simulink model "ActiveBrakeSystem"  (R2024b)
settings: Solver=VariableStepAuto  StartTime=0.0  StopTime=10  RelTol=1e-2
undefined symbols (not defined in the file or in its folder): Kd, Ki, Kp
libraries: fl_lib x24, nesl_utility x6, spsPWMGeneratorDCDCLib x1
settings Model: Creator=byxde  LastModifiedBy=emira
settings SolverCC: ZeroCrossAlgorithm=Adaptive
settings DebuggingCC: MaskedZcDiagnostic=none  IgnoredZcDiagnostic=none
settings ExplorerConfigSet: InternalSimMechanicsExplorerSettings="<ExplorerConfiguration><canonicalview>default</canonicalview><AnimationSetting><BasePlaybackSpeed>1.0</BasePlaybackSpeed><PlaybackSpeedFactor>1.0</PlaybackSpeedFactor></AnimationSetting><TilePanel><TileInfo><Tiles Columns=\"1\" Count=\"1\" Rows=\"1\"><Column Weight=\"1\"/><Row Weight=\"1\"/><Tile Height=\"1\" Width=\"1\" X=\"0\" Y=\"0\"/></Tiles></TileInfo><SceneInfo><SceneViewer><BGColor><R>0.60000002384185791</R><G>0.60000002384185791</G><B>0.60000002384185791</B></BGColor><Camera><DoPerspective>off</DoPerspective><Position><X>0</X><Y>-0.659999966621398926</Y><Z>0.00999999977648308169</Z></Position><Center><X>0</X><Y>0.340000033378601074</Y><Z>0.00999999977648308169</Z></Center><Up><X>0</X><Y>-0</Y><Z>1</Z></Up><ViewLimDist>1</ViewLimDist><YLim>0.164846771590149488</YLim><XLim>0.309000012278556835</XLim></Camera></SceneViewer></SceneInfo></TilePanel><MechEditorPanel><Cameras/><GfxPanelCameraMap/><VideoCreator><PlaybackSpeedRatio>1.0</PlaybackSpeedRatio><FrameRate>30</FrameRate><VideoFormat>Motion JPEG AVI</VideoFormat><FrameSize>auto</FrameSize></VideoCreator></MechEditorPanel></ExplorerConfiguration>"

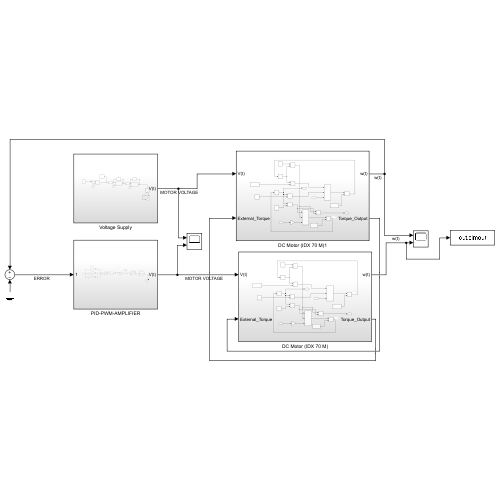
[thumbnail: Simulink's stored preview of the top-level diagram]
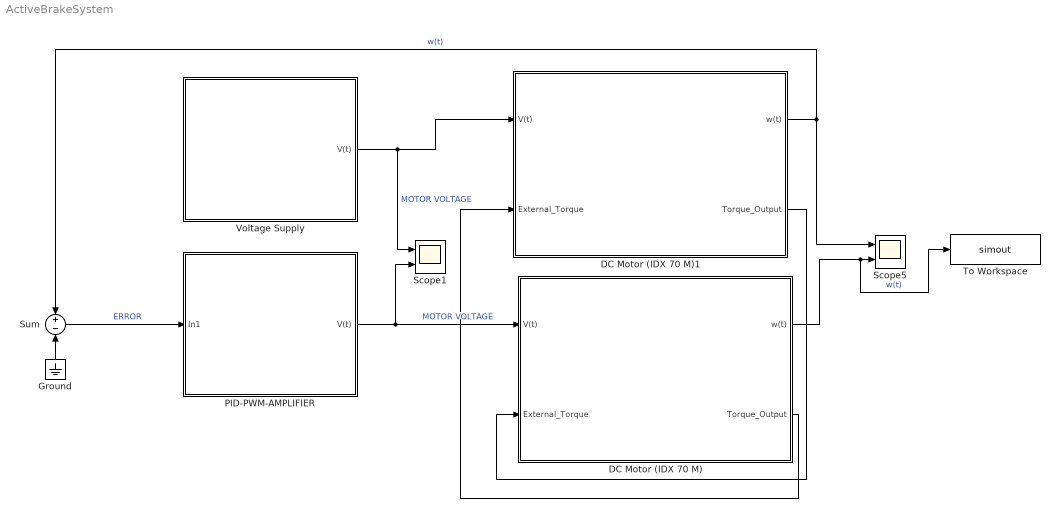
== system ActiveBrakeSystem ==
  DC Motor (IDX 70 M) : Subsystem
  DC Motor (IDX 70 M)1 : Subsystem
  Ground : Ground
  PID-PWM-AMPLIFIER : Subsystem
  Scope1 : Scope  NumInputPorts=2
  Scope5 : Scope  NumInputPorts=2
  Sum : Sum  Inputs=+-
  To Workspace : ToWorkspace  VariableName=simout  SaveFormat=Timeseries  SampleTime=-1
  Voltage Supply : Subsystem
  wires:
  DC Motor (IDX 70 M)/1(w(t)) -> To Workspace/1, Scope5/2  "w(t)"
  Sum/1 -> PID-PWM-AMPLIFIER/1(In1)  "ERROR"
  PID-PWM-AMPLIFIER/1(V(t)) -> Scope1/2, DC Motor (IDX 70 M)/1(V(t))  "MOTOR VOLTAGE"
  Ground/1 -> Sum/2
  DC Motor (IDX 70 M)1/1(w(t)) -> Sum/1, Scope5/1  "w(t)"
  DC Motor (IDX 70 M)1/2(Torque_Output) -> DC Motor (IDX 70 M)/2(External_Torque)
  DC Motor (IDX 70 M)/2(Torque_Output) -> DC Motor (IDX 70 M)1/2(External_Torque)
  Voltage Supply/1(V(t)) -> Scope1/1, DC Motor (IDX 70 M)1/1(V(t))  "MOTOR VOLTAGE"

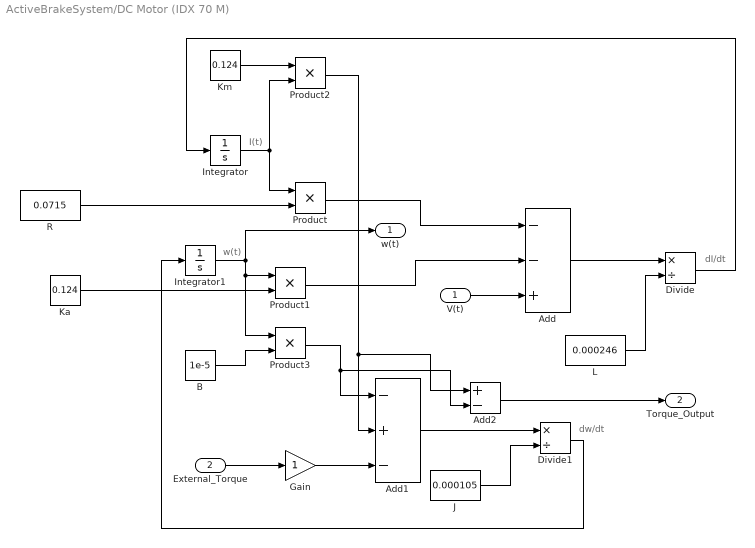
== system ActiveBrakeSystem/DC Motor (IDX 70 M) ==
  note: I(t)
  note: w(t)
  note: dI/dt
  note: dw/dt
  V(t) : Inport
  External_Torque : Inport  Port=2
  Add : Sum  Inputs=--+
  Add1 : Sum  Inputs=-+-
  Add2 : Sum  Inputs=+-
  B : Constant  Value=1e-5
  Divide : Product  Inputs=*/
  Divide1 : Product  Inputs=*/
  Gain : Gain
  Integrator : Integrator
  Integrator1 : Integrator  LimitOutput=on  UpperSaturationLimit=419  LowerSaturationLimit=-419
  J : Constant  Value=0.000105
  Ka : Constant  Value=0.124
  Km : Constant  Value=0.124
  L : Constant  Value=0.000246
  Product{,1..3} (4 alike) : Product
  R : Constant  Value=0.0715
  w(t) : Outport
  Torque_Output : Outport  Port=2
  wires:
  Integrator/1 -> Product2/2, Product/1
  J/1 -> Divide1/2
  Integrator1/1 -> w(t)/1, Product3/1, Product1/1
  Product3/1 -> Add2/2, Add1/1
  Product1/1 -> Add/2
  Product2/1 -> Add2/1, Add1/2
  Divide1/1 -> Integrator1/1
  R/1 -> Product/2
  L/1 -> Divide/2
  B/1 -> Product3/2
  Add1/1 -> Divide1/1
  Km/1 -> Product2/1
  Ka/1 -> Product1/2
  Product/1 -> Add/1
  Add/1 -> Divide/1
  Divide/1 -> Integrator/1
  V(t)/1 -> Add/3
  External_Torque/1 -> Gain/1
  Add2/1 -> Torque_Output/1
  Gain/1 -> Add1/3

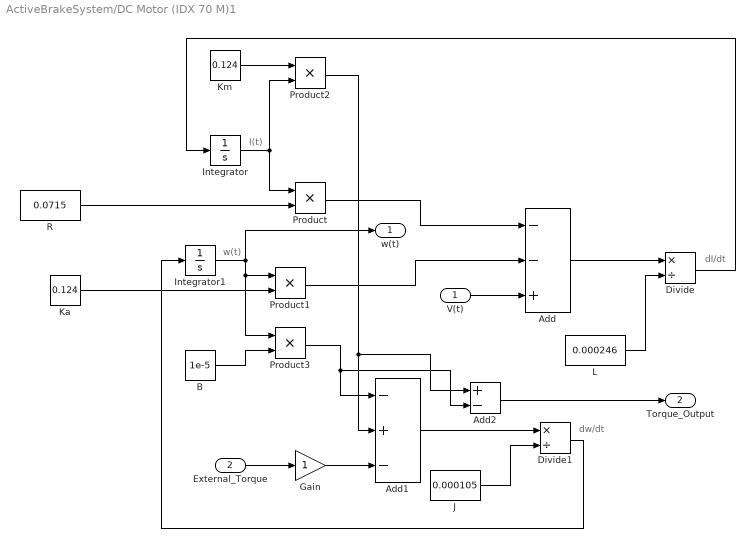
== system ActiveBrakeSystem/DC Motor (IDX 70 M)1 ==
  note: I(t)
  note: w(t)
  note: dI/dt
  note: dw/dt
  V(t) : Inport
  External_Torque : Inport  Port=2
  Add : Sum  Inputs=--+
  Add1 : Sum  Inputs=-+-
  Add2 : Sum  Inputs=+-
  B : Constant  Value=1e-5
  Divide : Product  Inputs=*/
  Divide1 : Product  Inputs=*/
  Gain : Gain
  Integrator : Integrator
  Integrator1 : Integrator  LimitOutput=on  UpperSaturationLimit=419  LowerSaturationLimit=-419
  J : Constant  Value=0.000105
  Ka : Constant  Value=0.124
  Km : Constant  Value=0.124
  L : Constant  Value=0.000246
  Product{,1..3} (4 alike) : Product
  R : Constant  Value=0.0715
  w(t) : Outport
  Torque_Output : Outport  Port=2
  wires:
  Integrator/1 -> Product2/2, Product/1
  J/1 -> Divide1/2
  Integrator1/1 -> w(t)/1, Product3/1, Product1/1
  Product3/1 -> Add2/2, Add1/1
  Product1/1 -> Add/2
  Product2/1 -> Add2/1, Add1/2
  Divide1/1 -> Integrator1/1
  R/1 -> Product/2
  L/1 -> Divide/2
  B/1 -> Product3/2
  Add1/1 -> Divide1/1
  Km/1 -> Product2/1
  Ka/1 -> Product1/2
  Product/1 -> Add/1
  Add/1 -> Divide/1
  Divide/1 -> Integrator/1
  V(t)/1 -> Add/3
  External_Torque/1 -> Gain/1
  Add2/1 -> Torque_Output/1
  Gain/1 -> Add1/3

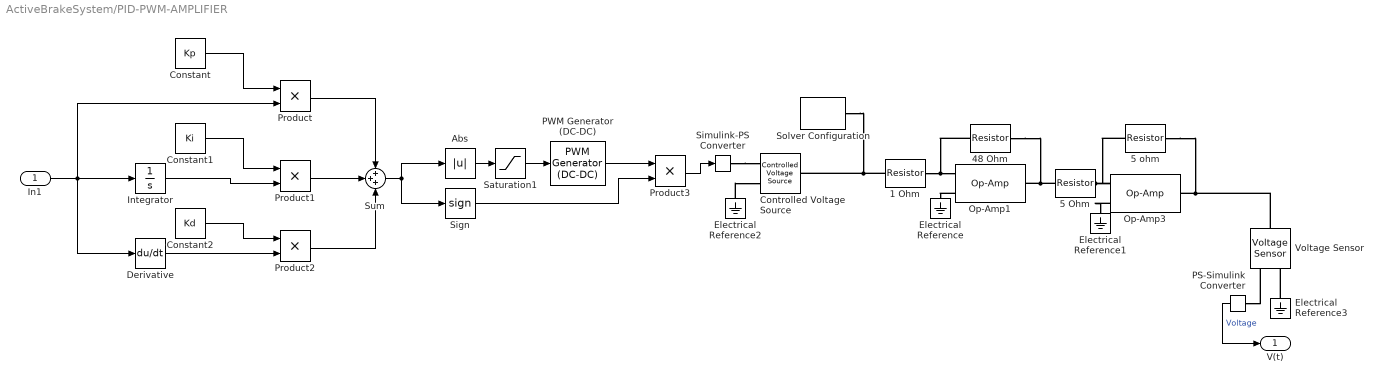
== system ActiveBrakeSystem/PID-PWM-AMPLIFIER ==
  In1 : Inport
  1 Ohm : fl_lib/Electrical/Electrical Elements/Resistor  R=1 Ohm  i_specify=off  i_priority=None  i=0 A  i_nominal_specify=off  i_nominal_value=1  i_nominal_unit=A  v_specify=off  v_priority=None  v=0 V  v_nominal_specify=off  v_nominal_value=1  v_nominal_unit=V
  48 Ohm : fl_lib/Electrical/Electrical Elements/Resistor  R=48 Ohm  i_specify=off  i_priority=None  i=0 A  i_nominal_specify=off  i_nominal_value=1  i_nominal_unit=A  v_specify=off  v_priority=None  v=0 V  v_nominal_specify=off  v_nominal_value=1  v_nominal_unit=V
  5 Ohm : fl_lib/Electrical/Electrical Elements/Resistor  R=5 Ohm  i_specify=off  i_priority=None  i=0 A  i_nominal_specify=off  i_nominal_value=1  i_nominal_unit=A  v_specify=off  v_priority=None  v=0 V  v_nominal_specify=off  v_nominal_value=1  v_nominal_unit=V
  5 ohm : fl_lib/Electrical/Electrical Elements/Resistor  R=5 Ohm  i_specify=off  i_priority=None  i=0 A  i_nominal_specify=off  i_nominal_value=1  i_nominal_unit=A  v_specify=off  v_priority=None  v=0 V  v_nominal_specify=off  v_nominal_value=1  v_nominal_unit=V
  Abs : Abs  SaturateOnIntegerOverflow=off
  Constant : Constant  Value=Kp
  Constant1 : Constant  Value=Ki
  Constant2 : Constant  Value=Kd
  Controlled Voltage Source : fl_lib/Electrical/Electrical Sources/Controlled Voltage Source
  Derivative : Derivative
  Electrical Reference{,1..3} (4 alike) : fl_lib/Electrical/Electrical Elements/Electrical Reference
  Integrator : Integrator
  Op-Amp1 : fl_lib/Electrical/Electrical Elements/Op-Amp  outI_specify=off  outI_priority=None  outI=0 A  outI_nominal_specify=off  outI_nominal_value=1  outI_nominal_unit=A
  Op-Amp3 : fl_lib/Electrical/Electrical Elements/Op-Amp  outI_specify=off  outI_priority=None  outI=0 A  outI_nominal_specify=off  outI_nominal_value=1  outI_nominal_unit=A
  PS-Simulink Converter : nesl_utility/PS-Simulink Converter  PhysicalDomain=network_engine_domain  SubClassName=ps_output  LeftPortType=input  RightPortType=output  PseudoPeriodic=off  Frequencies=[]  VectorFormat=inherit  Unit=inherit  AffineConversion=off
  PWM Generator (DC-DC) : spsPWMGeneratorDCDCLib/PWM Generator (DC-DC)  Fsw=100  Ts=0
  Product{,1..3} (4 alike) : Product
  Saturation1 : Saturate  UpperLimit=1  LowerLimit=0
  Sign : Signum
  Simulink-PS Converter : nesl_utility/Simulink-PS Converter  PhysicalDomain=network_engine_domain  SubClassName=ps_input  LeftPortType=input  RightPortType=output  PseudoPeriodic=off  Frequencies=[]  NoiseDistribution=none  NoiseParameters=[]  Unit=1  AffineConversion=off  FilteringAndDerivatives=provide  SimscapeFilterOrder=1  InputFilterTimeConstant=0.001  UdotUserProvided=0
  Solver Configuration : nesl_utility/Solver Configuration  PhysicalDomain=network_engine_domain  SubClassName=solver  LeftPortType=input  RightPortType=generic  Tones=[]  Harmonics=[]  SimulateNoise=off  Profile=off  UseLocalSampling=off  EnableSwitchedLinearOptims=on  FrequencyDomain=off  UseCCode=off  RelTol=0.001  AbsTol=0.001  MinStep=1e-09  ToWorkspace=off  RevertToSquareIcSolve=off  NumHomotopyIterations=100  PhasorMode=off  PhasorModeNumHarmonics=1  ConsistencySolver=NEWTON_XTOL_AFTER_FTOL  IndexReductionMethod=DerivativeReplacement  DoDC=off  ResidualTolerance=1e-09  ConsistencyTolSource=GLOBAL  ConsistencyAbsTol=0.001  ConsistencyRelTol=0.001  ConsistencyTolFactor=0.001  UseLocalSolver=off  LocalSolverChoice=NE_BACKWARD_EULER_ADVANCER  ResolveIndetEquations=on  FunctionEvalNumThread=1  LocalSolverSampleTime=0.001  DoFixedCost=off  MaxNonlinIter=3  MaxModeIter=2  ComputeImpulses=off  ImpulseIterations=2  LinearAlgebra=auto  LinearAlgebraNumThread=0  EquationFormulation=NE_TIME_EF  DelaysMemoryBudget=1024  AutomaticFiltering=on  FilteringTimeConstant=0.001  PartitionStorageMethod=AS_NEEDED  PartitionMemoryBudget=1024  PartitionMethod=ROBUST  MultibodyUseLocalSolver=off  MultibodyLocalSolverChoice=ODE1  MultibodyLocalSolverSampleTime=0.001
  Sum : Sum  Inputs=+++
  Voltage Sensor : fl_lib/Electrical/Electrical Sensors/Voltage Sensor
  V(t) : Outport
  wires:
  Derivative/1 -> Product2/2
  PS-Simulink Converter/1 -> V(t)/1  "Voltage"
  Product2/1 -> Sum/3
  Product/1 -> Sum/1
  Product3/1 -> Simulink-PS Converter/1
  Integrator/1 -> Product1/2
  Product1/1 -> Sum/2
  In1/1 -> Derivative/1, Integrator/1, Product/2
  Constant/1 -> Product/1
  Constant1/1 -> Product1/1
  Constant2/1 -> Product2/1
  Abs/1 -> Saturation1/1
  Sign/1 -> Product3/2
  PWM Generator (DC-DC)/1 -> Product3/1
  Sum/1 -> Sign/1, Abs/1
  Saturation1/1 -> PWM Generator (DC-DC)/1
  connections:
  1 Ohm/LConn1 -- Solver Configuration/RConn1 -- Controlled Voltage Source/LConn1
  Voltage Sensor/LConn1 -- 5 ohm/RConn1 -- Op-Amp3/RConn1
  Op-Amp1/RConn1 -- 48 Ohm/RConn1 -- 5 Ohm/LConn1
  Op-Amp3/LConn2 -- 5 Ohm/RConn1 -- 5 ohm/LConn1
  Op-Amp1/LConn2 -- 1 Ohm/RConn1 -- 48 Ohm/LConn1
  Electrical Reference2/LConn1 -- Controlled Voltage Source/RConn2
  Simulink-PS Converter/RConn1 -- Controlled Voltage Source/RConn1
  Electrical Reference3/LConn1 -- Voltage Sensor/RConn2
  PS-Simulink Converter/LConn1 -- Voltage Sensor/RConn1
  Op-Amp3/LConn1 -- Electrical Reference1/LConn1
  Op-Amp1/LConn1 -- Electrical Reference/LConn1

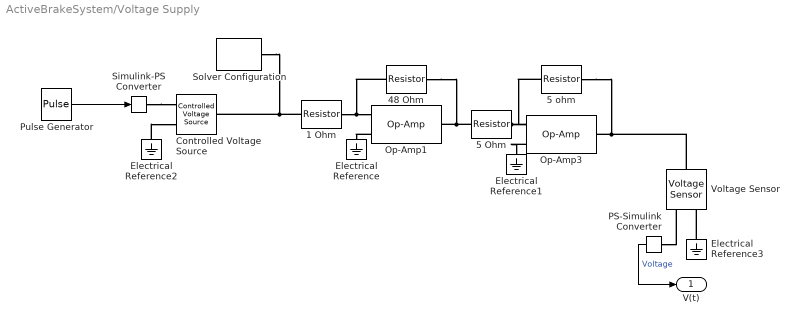
== system ActiveBrakeSystem/Voltage Supply ==
  1 Ohm : fl_lib/Electrical/Electrical Elements/Resistor  R=1 Ohm  i_specify=off  i_priority=None  i=0 A  i_nominal_specify=off  i_nominal_value=1  i_nominal_unit=A  v_specify=off  v_priority=None  v=0 V  v_nominal_specify=off  v_nominal_value=1  v_nominal_unit=V
  48 Ohm : fl_lib/Electrical/Electrical Elements/Resistor  R=48 Ohm  i_specify=off  i_priority=None  i=0 A  i_nominal_specify=off  i_nominal_value=1  i_nominal_unit=A  v_specify=off  v_priority=None  v=0 V  v_nominal_specify=off  v_nominal_value=1  v_nominal_unit=V
  5 Ohm : fl_lib/Electrical/Electrical Elements/Resistor  R=5 Ohm  i_specify=off  i_priority=None  i=0 A  i_nominal_specify=off  i_nominal_value=1  i_nominal_unit=A  v_specify=off  v_priority=None  v=0 V  v_nominal_specify=off  v_nominal_value=1  v_nominal_unit=V
  5 ohm : fl_lib/Electrical/Electrical Elements/Resistor  R=5 Ohm  i_specify=off  i_priority=None  i=0 A  i_nominal_specify=off  i_nominal_value=1  i_nominal_unit=A  v_specify=off  v_priority=None  v=0 V  v_nominal_specify=off  v_nominal_value=1  v_nominal_unit=V
  Controlled Voltage Source : fl_lib/Electrical/Electrical Sources/Controlled Voltage Source
  Electrical Reference{,1..3} (4 alike) : fl_lib/Electrical/Electrical Elements/Electrical Reference
  Op-Amp1 : fl_lib/Electrical/Electrical Elements/Op-Amp  outI_specify=off  outI_priority=None  outI=0 A  outI_nominal_specify=off  outI_nominal_value=1  outI_nominal_unit=A
  Op-Amp3 : fl_lib/Electrical/Electrical Elements/Op-Amp  outI_specify=off  outI_priority=None  outI=0 A  outI_nominal_specify=off  outI_nominal_value=1  outI_nominal_unit=A
  PS-Simulink Converter : nesl_utility/PS-Simulink Converter  PhysicalDomain=network_engine_domain  SubClassName=ps_output  LeftPortType=input  RightPortType=output  PseudoPeriodic=off  Frequencies=[]  VectorFormat=inherit  Unit=inherit  AffineConversion=off
  Pulse Generator : DiscretePulseGenerator  PulseType=Time based  Period=1/50000  PulseWidth=99
  Simulink-PS Converter : nesl_utility/Simulink-PS Converter  PhysicalDomain=network_engine_domain  SubClassName=ps_input  LeftPortType=input  RightPortType=output  PseudoPeriodic=off  Frequencies=[]  NoiseDistribution=none  NoiseParameters=[]  Unit=1  AffineConversion=off  FilteringAndDerivatives=provide  SimscapeFilterOrder=1  InputFilterTimeConstant=0.001  UdotUserProvided=0
  Solver Configuration : nesl_utility/Solver Configuration  PhysicalDomain=network_engine_domain  SubClassName=solver  LeftPortType=input  RightPortType=generic  Tones=[]  Harmonics=[]  SimulateNoise=off  Profile=off  UseLocalSampling=off  EnableSwitchedLinearOptims=on  FrequencyDomain=off  UseCCode=off  RelTol=0.001  AbsTol=0.001  MinStep=1e-09  ToWorkspace=off  RevertToSquareIcSolve=off  NumHomotopyIterations=100  PhasorMode=off  PhasorModeNumHarmonics=1  ConsistencySolver=NEWTON_XTOL_AFTER_FTOL  IndexReductionMethod=DerivativeReplacement  DoDC=off  ResidualTolerance=1e-09  ConsistencyTolSource=GLOBAL  ConsistencyAbsTol=0.001  ConsistencyRelTol=0.001  ConsistencyTolFactor=0.001  UseLocalSolver=off  LocalSolverChoice=NE_BACKWARD_EULER_ADVANCER  ResolveIndetEquations=on  FunctionEvalNumThread=1  LocalSolverSampleTime=0.001  DoFixedCost=off  MaxNonlinIter=3  MaxModeIter=2  ComputeImpulses=off  ImpulseIterations=2  LinearAlgebra=auto  LinearAlgebraNumThread=0  EquationFormulation=NE_TIME_EF  DelaysMemoryBudget=1024  AutomaticFiltering=on  FilteringTimeConstant=0.001  PartitionStorageMethod=AS_NEEDED  PartitionMemoryBudget=1024  PartitionMethod=ROBUST  MultibodyUseLocalSolver=off  MultibodyLocalSolverChoice=ODE1  MultibodyLocalSolverSampleTime=0.001
  Voltage Sensor : fl_lib/Electrical/Electrical Sensors/Voltage Sensor
  V(t) : Outport
  wires:
  PS-Simulink Converter/1 -> V(t)/1  "Voltage"
  Pulse Generator/1 -> Simulink-PS Converter/1
  connections:
  1 Ohm/LConn1 -- Solver Configuration/RConn1 -- Controlled Voltage Source/LConn1
  Voltage Sensor/LConn1 -- 5 ohm/RConn1 -- Op-Amp3/RConn1
  Op-Amp1/RConn1 -- 48 Ohm/RConn1 -- 5 Ohm/LConn1
  Op-Amp3/LConn2 -- 5 Ohm/RConn1 -- 5 ohm/LConn1
  Op-Amp1/LConn2 -- 1 Ohm/RConn1 -- 48 Ohm/LConn1
  Electrical Reference2/LConn1 -- Controlled Voltage Source/RConn2
  Simulink-PS Converter/RConn1 -- Controlled Voltage Source/RConn1
  Electrical Reference3/LConn1 -- Voltage Sensor/RConn2
  PS-Simulink Converter/LConn1 -- Voltage Sensor/RConn1
  Op-Amp3/LConn1 -- Electrical Reference1/LConn1
  Op-Amp1/LConn1 -- Electrical Reference/LConn1
